simulink model "measurement_sim"  (R2023b)
settings: Solver=FixedStepAuto  StartTime=0.0  StopTime=36000  FixedStep=1/30  RelTol=1e-8
undefined symbols (not defined in the file or in its folder): DiscIntNeverNeededParam, IMU, MainSpacecraft
libraries: vrlib x2, dyn_lib x1, nav_lib x1
settings Model: DataDictionary=SimulationDict.sldd  EnableAccessToBaseWorkspace=off  SimulationMode=accelerator  Creator=brent  LastModifiedBy=brent

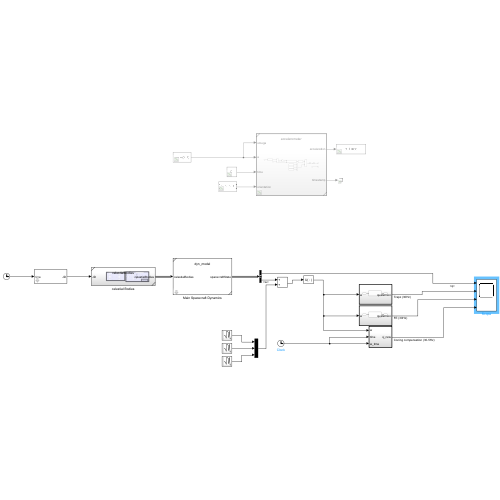
[thumbnail: Simulink's stored preview of the top-level diagram]
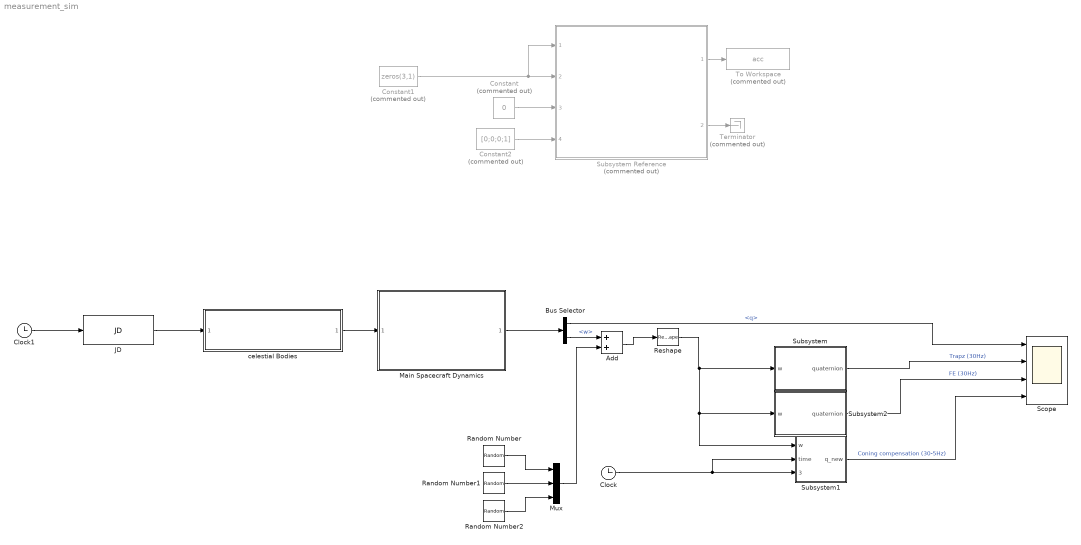
== system measurement_sim ==
  Add : Sum
  Bus Selector : BusSelector  OutputSignals=q,w
  Clock : Clock
  Clock1 : Clock
  Constant : Constant  Commented=on  Value=0
  Constant1 : Constant  Commented=on  Value=zeros(3,1)
  Constant2 : Constant  Commented=on  Value=[0;0;0;1]
  JD : dyn_lib/JD  year=Environment.Date.year  month=Environment.Date.month  day=Environment.Date.day  hour=Environment.Date.hour  min=Environment.Date.min  sec=Environment.Date.sec
      settings: SourceProductName=Dynamics library
  Main Spacecraft Dynamics : Subsystem  ReferencedSubsystem=dyn_model  Environment=Environment  Spacecraft=MainSpacecraft  sc_type="\"main\""
  Mux : Mux  Inputs=3
  Random Number : RandomNumber  Variance=(0.001*pi/180)^2  Seed=5638
  Random Number1 : RandomNumber  Variance=(0.001*pi/180)^2  Seed=3456
  Random Number2 : RandomNumber  Variance=(0.001*pi/180)^2  Seed=760
  Reshape : Reshape
  Scope : Scope  NumInputPorts=4
  Subsystem : Subsystem  TreatAsAtomicUnit=on  SystemSampleTime=1/30
  Subsystem Reference : Subsystem  Commented=on  TreatAsAtomicUnit=on  SystemSampleTime=IMU.accelerometer.sampleTime.value  ReferencedSubsystem=accelerometer
  Subsystem1 : Subsystem  TreatAsAtomicUnit=on  SystemSampleTime=1/30
  Subsystem2 : Subsystem  TreatAsAtomicUnit=on  SystemSampleTime=1/30
  Terminator : Terminator  Commented=on
  To Workspace : ToWorkspace  Commented=on  VariableName=acc  SampleTime=-1
      settings: Save2DSignal=2-D array (concatenate along first dimension)
  celestial Bodies : Subsystem  ReferencedSubsystem=celestialBodies
      settings: PermitHierarchicalResolution=None
  wires:
  Constant/1 -> Subsystem Reference/3
  Constant1/1 -> Subsystem Reference/1, Subsystem Reference/2
  Constant2/1 -> Subsystem Reference/4
  Subsystem Reference/2 -> Terminator/1
  Subsystem Reference/1 -> To Workspace/1
  Clock/1 -> Subsystem1/2(time), Subsystem1/3(w_time)
  Bus Selector/1 -> Scope/1  "<q>"
  Clock1/1 -> JD/1
  celestial Bodies/1 -> Main Spacecraft Dynamics/1
  JD/1 -> celestial Bodies/1
  Main Spacecraft Dynamics/1 -> Bus Selector/1
  Subsystem/1(quaternion) -> Scope/2  "Trapz (30Hz)"
  Subsystem1/1(q_new) -> Scope/4  "Coning compensation (30-5Hz)"
  Subsystem2/1(quaternion) -> Scope/3  "FE (30Hz)"
  Reshape/1 -> Subsystem2/1(w), Subsystem1/1(w), Subsystem/1(w)
  Bus Selector/2 -> Add/1  "<w>"
  Add/1 -> Reshape/1
  Mux/1 -> Add/2
  Random Number/1 -> Mux/1
  Random Number1/1 -> Mux/2
  Random Number2/1 -> Mux/3

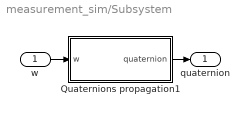
== system measurement_sim/Subsystem ==
  w : Inport
  Quaternions propagation1 : Subsystem  AncestorBlock=dyn_lib/Quaternions propagation  mask{q0=MainSpacecraft.q0.value}
      mask prompts: q0 "Initial attitude quaternion"
      mask DialogControl DescGroupVar Prompt: Quaternion propagation
  quaternion : Outport
  wires:
  w/1 -> Quaternions propagation1/1(w)
  Quaternions propagation1/1(quaternion) -> quaternion/1

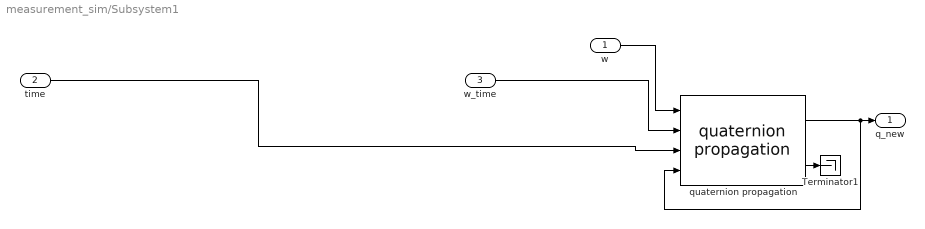
== system measurement_sim/Subsystem1 ==
  w : Inport
  time : Inport  Port=2
  w_time : Inport  Port=3
  Terminator1 : Terminator
  quaternion propagation : nav_lib/quaternion propagation  N=6  q0=MainSpacecraft.q0.value
      settings: SourceProductName=Navigation library
  q_new : Outport
  wires:
  quaternion propagation/2 -> Terminator1/1
  time/1 -> quaternion propagation/3
  quaternion propagation/1 -> quaternion propagation/4, q_new/1
  w_time/1 -> quaternion propagation/2
  w/1 -> quaternion propagation/1

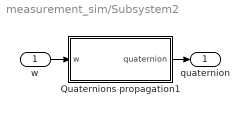
== system measurement_sim/Subsystem2 ==
  w : Inport
  Quaternions propagation1 : Subsystem  AncestorBlock=dyn_lib/Quaternions propagation  mask{q0=MainSpacecraft.q0.value}
      mask prompts: q0 "Initial attitude quaternion"
      mask DialogControl DescGroupVar Prompt: Quaternion propagation
  quaternion : Outport
  wires:
  Quaternions propagation1/1(quaternion) -> quaternion/1
  w/1 -> Quaternions propagation1/1(w)

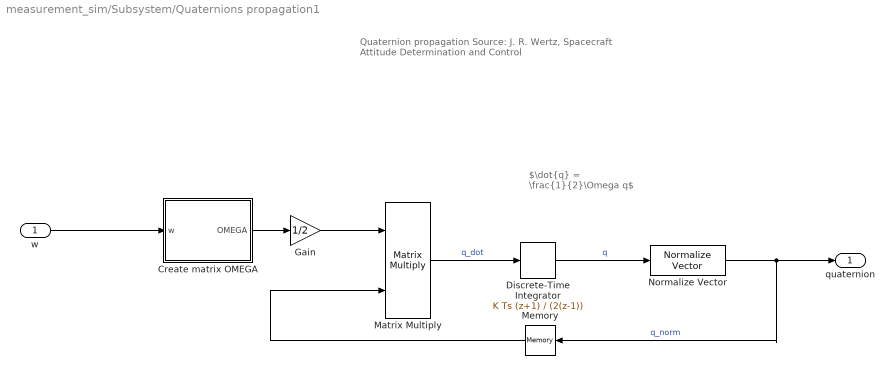
== system measurement_sim/Subsystem/Quaternions propagation1 ==
  note: $\dot{q} = \frac{1}{2}\Omega q$
  note: Quaternion propagation
      |
      | Source:
      | J. R. Wertz, Spacecraft Attitude Determination and Control
  w : Inport
  Create matrix OMEGA : Subsystem
  Discrete-Time Integrator : DiscreteIntegrator  IntegratorMethod=Integration: Trapezoidal  InitialCondition=q0  SampleTime=-1  ICPrevOutput=DiscIntNeverNeededParam  ICPrevScaledInput=DiscIntNeverNeededParam
  Gain : Gain  Gain=1/2  SaturateOnIntegerOverflow=on  OutDataTypeStr=Inherit: Same as input  ParamDataTypeStr=Inherit: Same as input
  Matrix Multiply : Product  Multiplication=Matrix(*)
  Memory : Memory  InitialCondition=q0  InheritSampleTime=on
  Normalize Vector : vrlib/Utilities/Normalize Vector  maxzero=0
  quaternion : Outport
  wires:
  w/1 -> Create matrix OMEGA/1(w)
  Matrix Multiply/1 -> Discrete-Time Integrator/1  "q_dot"
  Normalize Vector/1 -> quaternion/1, Memory/1  "q_norm"
  Discrete-Time Integrator/1 -> Normalize Vector/1  "q"
  Create matrix OMEGA/1(OMEGA) -> Gain/1
  Gain/1 -> Matrix Multiply/1
  Memory/1 -> Matrix Multiply/2

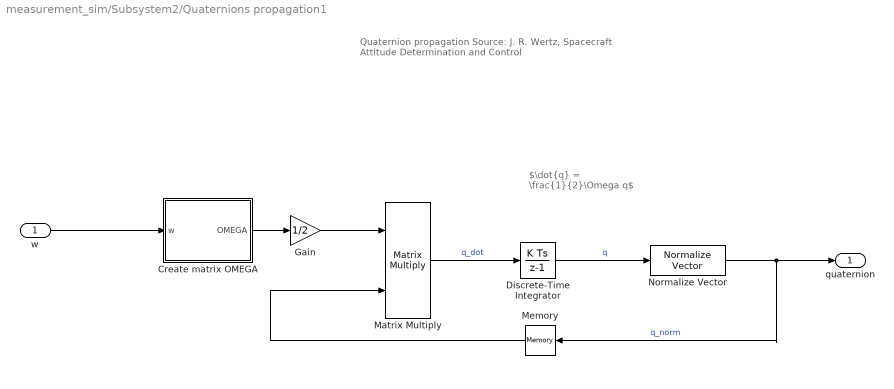
== system measurement_sim/Subsystem2/Quaternions propagation1 ==
  note: Quaternion propagation
      |
      | Source:
      | J. R. Wertz, Spacecraft Attitude Determination and Control
  note: $\dot{q} = \frac{1}{2}\Omega q$
  w : Inport
  Create matrix OMEGA : Subsystem
  Discrete-Time Integrator : DiscreteIntegrator  InitialCondition=q0  SampleTime=-1  ICPrevOutput=DiscIntNeverNeededParam  ICPrevScaledInput=DiscIntNeverNeededParam
  Gain : Gain  Gain=1/2  SaturateOnIntegerOverflow=on  OutDataTypeStr=Inherit: Same as input  ParamDataTypeStr=Inherit: Same as input
  Matrix Multiply : Product  Multiplication=Matrix(*)
  Memory : Memory  InitialCondition=q0  InheritSampleTime=on
  Normalize Vector : vrlib/Utilities/Normalize Vector  maxzero=0
  quaternion : Outport
  wires:
  Memory/1 -> Matrix Multiply/2
  Gain/1 -> Matrix Multiply/1
  Create matrix OMEGA/1(OMEGA) -> Gain/1
  Discrete-Time Integrator/1 -> Normalize Vector/1  "q"
  Normalize Vector/1 -> Memory/1, quaternion/1  "q_norm"
  Matrix Multiply/1 -> Discrete-Time Integrator/1  "q_dot"
  w/1 -> Create matrix OMEGA/1(w)

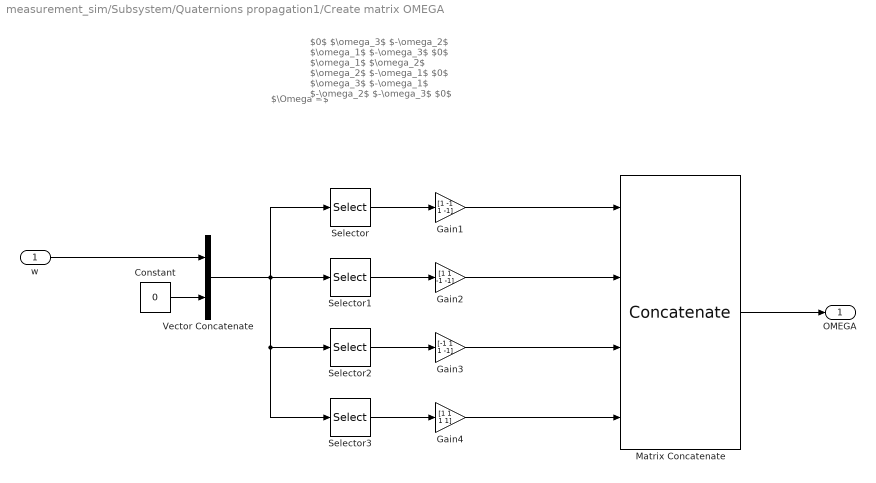
== system measurement_sim/Subsystem/Quaternions propagation1/Create matrix OMEGA ==
  note: $\Omega =$
  note: $0$
      | $\omega_3$
      | $-\omega_2$
      | $\omega_1$
      |
      | $-\omega_3$
      | $0$
      | $\omega_1$
      | $\omega_2$
      |
      | $\omega_2$
      | $-\omega_1$
      | $0$
      | $\omega_3$
      |
      | $-\omega_1$
      | $-\omega_2$
      | $-\omega_3$
      | $0$
  w : Inport
  Constant : Constant  Value=0
  Gain1 : Gain  Gain=[1 -1 1 -1]
  Gain2 : Gain  Gain=[1 1 -1 -1]
  Gain3 : Gain  Gain=[-1 1 1 -1]
  Gain4 : Gain  Gain=[1 1 1 1]
  Matrix Concatenate : Concatenate  NumInputs=4  Mode=Multidimensional array  ConcatenateDimension=2
  Selector : Selector  InputPortWidth=4  IndexOptions=Index vector (dialog)  Indices=[4 3 2 1]  OutputSizes=1
  Selector1 : Selector  InputPortWidth=4  IndexOptions=Index vector (dialog)  Indices=[3 4 1 2]  OutputSizes=1
  Selector2 : Selector  InputPortWidth=4  IndexOptions=Index vector (dialog)  Indices=[2 1 4 3]  OutputSizes=1
  Selector3 : Selector  InputPortWidth=4  IndexOptions=Index vector (dialog)  Indices=[1 2 3 4]  OutputSizes=1
  Vector Concatenate : Concatenate
  OMEGA : Outport
  wires:
  Selector/1 -> Gain1/1
  Selector2/1 -> Gain3/1
  Selector3/1 -> Gain4/1
  Vector Concatenate/1 -> Selector/1, Selector1/1, Selector3/1, Selector2/1
  Constant/1 -> Vector Concatenate/2
  Selector1/1 -> Gain2/1
  Matrix Concatenate/1 -> OMEGA/1
  w/1 -> Vector Concatenate/1
  Gain1/1 -> Matrix Concatenate/1
  Gain2/1 -> Matrix Concatenate/2
  Gain3/1 -> Matrix Concatenate/3
  Gain4/1 -> Matrix Concatenate/4

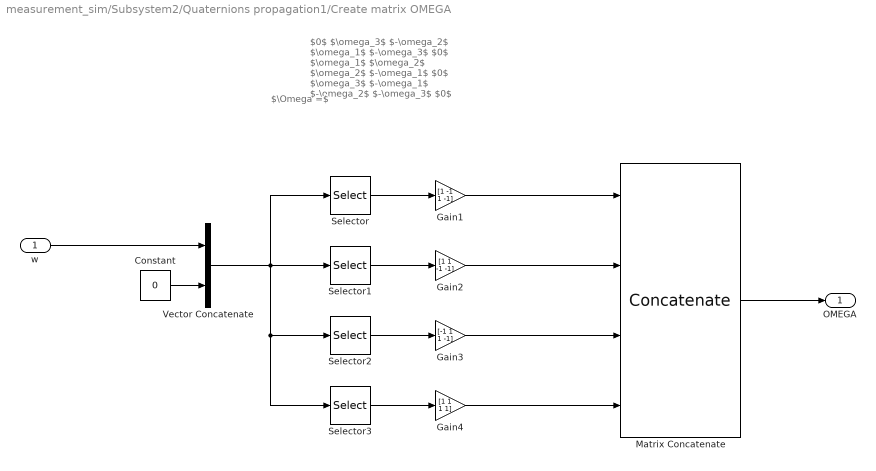
== system measurement_sim/Subsystem2/Quaternions propagation1/Create matrix OMEGA ==
  note: $0$
      | $\omega_3$
      | $-\omega_2$
      | $\omega_1$
      |
      | $-\omega_3$
      | $0$
      | $\omega_1$
      | $\omega_2$
      |
      | $\omega_2$
      | $-\omega_1$
      | $0$
      | $\omega_3$
      |
      | $-\omega_1$
      | $-\omega_2$
      | $-\omega_3$
      | $0$
  note: $\Omega =$
  w : Inport
  Constant : Constant  Value=0
  Gain1 : Gain  Gain=[1 -1 1 -1]
  Gain2 : Gain  Gain=[1 1 -1 -1]
  Gain3 : Gain  Gain=[-1 1 1 -1]
  Gain4 : Gain  Gain=[1 1 1 1]
  Matrix Concatenate : Concatenate  NumInputs=4  Mode=Multidimensional array  ConcatenateDimension=2
  Selector : Selector  InputPortWidth=4  IndexOptions=Index vector (dialog)  Indices=[4 3 2 1]  OutputSizes=1
  Selector1 : Selector  InputPortWidth=4  IndexOptions=Index vector (dialog)  Indices=[3 4 1 2]  OutputSizes=1
  Selector2 : Selector  InputPortWidth=4  IndexOptions=Index vector (dialog)  Indices=[2 1 4 3]  OutputSizes=1
  Selector3 : Selector  InputPortWidth=4  IndexOptions=Index vector (dialog)  Indices=[1 2 3 4]  OutputSizes=1
  Vector Concatenate : Concatenate
  OMEGA : Outport
  wires:
  Gain4/1 -> Matrix Concatenate/4
  Gain3/1 -> Matrix Concatenate/3
  Gain2/1 -> Matrix Concatenate/2
  Gain1/1 -> Matrix Concatenate/1
  w/1 -> Vector Concatenate/1
  Matrix Concatenate/1 -> OMEGA/1
  Selector1/1 -> Gain2/1
  Constant/1 -> Vector Concatenate/2
  Vector Concatenate/1 -> Selector2/1, Selector3/1, Selector1/1, Selector/1
  Selector3/1 -> Gain4/1
  Selector2/1 -> Gain3/1
  Selector/1 -> Gain1/1
